simulink model "TASK3_LAB"  (R2024b)
settings: Solver=ode4  StartTime=0.0  StopTime=T_SIM  FixedStep=T_s  RelTol=1e-3
values from neighbouring files (symbols this model uses):
  control_par = [1.5, 1.5, 0.3]    [TASK1_Script.m]    (also in TASK2_LAB_SCRIPT.m = update_control_par(controller_index); TASK2_Scirpt.m = [k1, k2,b]; TASK3_Script.m = update_control_par(controller_index))
  controller_index = 2    [TASK2_LAB_SCRIPT.m]    (also in TASK2_Scirpt.m = 3; TASK3_Script.m = 3)
  d = d_actual    (= 0.1604)    [TASK1_Script.m]    (also in TASK2_LAB_SCRIPT.m; TASK2_Scirpt.m; TASK3_Script.m)
  D = diag([0.8e-3, 0.8e-3, 5e-3, 0.0175/6, 0.0175/6, 0.0175/6*T_s, 0.0175/6*T_s].^2)    [TASK1_Script.m]    (also in TASK2_LAB_SCRIPT.m; TASK2_Scirpt.m; TASK3_Script.m)
  d_actual = 0.16040    (= 0.1604)    [TASK1_Script.m]    (also in TASK2_LAB_SCRIPT.m; TASK2_Scirpt.m; TASK3_Script.m)
  H_enc = [0, 0, 0, 1, 0, 0, 0 ... (first row only)    [TASK1_Script.m]    (also in TASK2_LAB_SCRIPT.m; TASK2_Scirpt.m; TASK3_Script.m)
  H_gyro = [0, 0, 0, 0, 0, -r_actual/d_actual, r_actual/d_actual]    [TASK1_Script.m]    (also in TASK2_LAB_SCRIPT.m; TASK2_Scirpt.m; TASK3_Script.m)
  H_motion_cap = [1, 0, 0, 0, 0, 0, 0 ... (first row only)    [TASK1_Script.m]    (also in TASK2_LAB_SCRIPT.m; TASK2_Scirpt.m; TASK3_Script.m)
  omega_M = 10    [TASK1_Script.m]    (also in TASK2_LAB_SCRIPT.m; TASK2_Scirpt.m; TASK3_Script.m)
  P_INIT_EKF = diag([0.1, 0.1, 0.2, 0.0175/6, 0.0175/6, 0.0175/6*T_s, 0.0175/6*T_s].^2)    [TASK1_Script.m]    (also in TASK2_LAB_SCRIPT.m; TASK2_Scirpt.m; TASK3_Script.m)
  PHI_INIT = [0;0]    [TASK1_Script.m]    (also in TASK2_LAB_SCRIPT.m; TASK2_Scirpt.m; TASK3_Script.m)
  Q_INIT = Q_INIT_4    [TASK1_Script.m]    (also in TASK2_LAB_SCRIPT.m = [-1.6;-1.1;0]; TASK2_Scirpt.m = [-1.6;-1.1;0]; TASK3_Script.m = % ARRIVO TASK 2)
  r = r_actual    (= 0.03293)    [TASK1_Script.m]    (also in TASK2_LAB_SCRIPT.m; TASK2_Scirpt.m; TASK3_Script.m)
  R_3 = diag(([sigma_motion_capture, sigma_motion_capture, sigma_motion_capture,               sigma_enc, sigma_enc, sigma_imu]).^2)    [TASK1_Script.m]    (also in TASK2_LAB_SCRIPT.m; TASK2_Scirpt.m; TASK3_Script.m)
  r_actual = 0.03293    [TASK1_Script.m]    (also in TASK2_LAB_SCRIPT.m; TASK2_Scirpt.m; TASK3_Script.m)
  T_s = 0.04    [TASK1_Script.m]    (also in TASK2_LAB_SCRIPT.m; TASK2_Scirpt.m; TASK3_Script.m; plot_4_wheel_velocities.m)
  Z_INIT_EKF = [Q_INIT; 0; 0; 0; 0]    [TASK1_Script.m]    (also in TASK2_LAB_SCRIPT.m; TASK2_Scirpt.m; TASK3_Script.m)
undefined symbols (not defined in the file or in its folder): p_loss, X, Y
libraries: robotlib x6, sharedtransform x2
(part 2 of 2)

== matlab function TASK3_LAB/Localizzazione EKF/MATLAB Function ==
  data: P_filt input; P_new output; z_filt input; z_new output; u input; y_new input; D parameter; T_s parameter; r_actual parameter; d_actual parameter; H_enc parameter; H_gyro parameter; H_motion_cap parameter; R_3 parameter; q_EKF output
function [P_new, z_new, q_EKF] = EKF_filtering(P_filt, z_filt, u, y_new, D, T_s, r_actual, d_actual, H_enc, H_gyro, H_motion_cap, R_3)

    % Def state z_filt: [xk , yk , thetak , delta_phi_L_km1 , delta_phi_R_km1 , wLk , wRk ]

    r = r_actual;
    d = d_actual;
        
    % Extraction variables
    x_k = z_filt(1);
    y_k = z_filt(2);
    theta_k = z_filt(3);
    delta_phi_L_km1 = z_filt(4);
    delta_phi_R_km1 = z_filt(5); 
    wL_k = z_filt(6);               % estimate wheels velocities
    wR_k = z_filt(7);
    
    uL_k = u(1);                    % actual wheels velocities (from command input v,w)
    uR_k = u(2);

    % ----------------------

    % PREDICT STEP
    v_k = (r/2) * (wL_k + wR_k);
    omega_k = (r/d) * (wR_k - wL_k);
    theta_mean = theta_k + (omega_k * T_s) / 2;
        
    % State Prediction (approximation with RK2)
    x_kp1 = x_k + v_k * T_s * cos(theta_mean);
    y_kp1 = y_k + v_k * T_s * sin(theta_mean);
    theta_kp1 = theta_k + omega_k * T_s;

    theta_kp1 = atan2(sin(theta_kp1), cos(theta_kp1));
    
    delta_phi_L_k = wL_k * T_s;
    delta_phi_R_k = wR_k * T_s;
    
    wL_kp1 = uL_k; 
    wR_kp1 = uR_k;
    
    z_hat = [x_kp1; y_kp1; theta_kp1; delta_phi_L_k; delta_phi_R_k; wL_kp1; wR_kp1];
    
    % F derivation
    F = zeros(7,7);
    
    F(1,1) = 1;
    F(1, 3) = -T_s * v_k * sin(theta_mean);
    F(1, 6) = (T_s * r / 2) * cos(theta_mean) - v_k * T_s * sin(theta_mean) * (-T_s * r / (2 * d));
    F(1, 7) = (T_s * r / 2) * cos(theta_mean) - v_k * T_s * sin(theta_mean) * (T_s * r / (2 * d));
    
    F(2,2) = 1;
    F(2, 3) = v_k * T_s * cos(theta_mean);
    F(2, 6) = (T_s * r / 2) * sin(theta_mean) + v_k * T_s * cos(theta_mean) * (-T_s * r / (2 * d));
    F(2, 7) = (T_s * r / 2) * sin(theta_mean) + v_k * T_s * cos(theta_mean) * (T_s * r / (2 * d));

    F(3,3) = 1;
    F(3, 6) = -T_s * r / d;
    F(3, 7) = T_s * r / d;

    F(4, 6) = T_s;
    F(5, 7) = T_s;
    
    % Covariance Prediction
    P_hat = F * P_filt * F' + D;
    
    % ----------------------

    % UPDATE STEP
    % H and R will depend on the measurement data y_new and Test_case

    % enc_values (delta_phi)
    % IMU_values (w_gyro)
    % Motion_capture (state q)

    % y_new = [x; y; theta; delta_phi_L; delta_phi_R; omega_gyro]

    %% OBSERVATION MATRIX H ALWAYS FULL (6X7) AND ALSO Y_NEW (6X1) 
    H_full = [H_motion_cap; H_enc; H_gyro];
    y_meas = y_new; 
    
    % Start with full matrix R_3 
    R_current = R_3;
    INFINITY_VAR = 1e9; % Infinite var to put down the Kalman gain

    % IMU not available
    R_current(6,6) = INFINITY_VAR;
    
    % TEST 3: all active, possibile data loss
    if any(isnan(y_new(1:3)))   
        y_meas(1:3) = 0;    % force to zero just for completness
        R_current(1,1) = INFINITY_VAR; 
        R_current(2,2) = INFINITY_VAR; 
        R_current(3,3) = INFINITY_VAR;
    end

    
    % Innovation e_pred
    y_hat = H_full * z_hat;
    e_kp1 = y_meas - y_hat;

    e_kp1(3) = atan2(sin(e_kp1(3)), cos(e_kp1(3)));
    
    % Kalman Gain K_pred
    K = P_hat * H_full' / (H_full * P_hat * H_full' + R_current);   
    
    % State and Covariance Update
    z_new = z_hat + K * e_kp1;

    z_new(3) = atan2(sin(z_new(3)), cos(z_new(3)));
    
    P_new = P_hat - K * H_full * P_hat;


    q_EKF = z_new(1:3);

end

== matlab function TASK3_LAB/Planning/Trajectory Planning ==
  data: t input; q_d output; dq_d output; u_DF output; T_trj parameter
function [q_d, dq_d, u_DF] = get_circualt_traj_TASK3(t, T_trj)
   
    % center
    x_c = 2.0;     % x10-x9 /2
    y_c = 0.0;

    % starting point (x8, y4) = (1.45, -0.30)
    x0 = 1.45;
    y0 = -0.30;

    % Raggio e angolo iniziale (calcolati dal punto di partenza)
    r = sqrt((x0 - x_c)^2 + (y0 - y_c)^2);
    phi0 = atan2(y0 - y_c, x0 - x_c);

    % 1.5 giri = 3*pi rad in T_trj secondi
    omega = 3 * pi / T_trj;   % constant ang vel
    theta_prime = omega*t;

    phi = phi0 + theta_prime;

    q_d = [x_c + r*cos(phi); y_c + r*sin(phi); phi + pi/2];
    
    dq_d = [-omega*r*sin(phi); omega*r*cos(phi); omega];

    u_DF = [omega*r; omega];
    
end
